simulink library "VariableOrderDifferentialEquationsToolbox"  (R2020a)
settings: Solver=VariableStepAuto  StartTime=0.0  StopTime=10.0  RelTol=1e-3
(part 3 of 3)

== matlab function VariableOrderDifferentialEquationsToolbox/GL FVOPID - Type A/integralErrorDependentSubsystem/Integral Error Depenent Order ==
  data: e input; y output; errorValuesVector input; orderValuesVector input
function y = integralOrderFunction(e, errorValuesVector, orderValuesVector)
    y = fvopidToolbox.utils.getOrderValue(e, errorValuesVector, orderValuesVector);
end

== matlab function VariableOrderDifferentialEquationsToolbox/GL FVOPID - Type A/derivativeRatioDependentSubsystem/Integral Error Depenent Order 2 ==
  data: e input; setpoint input; y output; errorValuesVector input; orderValuesVector input
function y = integralOrderFunction(e, setpoint, errorValuesVector, orderValuesVector)
    y = fvopidToolbox.utils.getOrderValue(e/setpoint, errorValuesVector, orderValuesVector);
end

== matlab function VariableOrderDifferentialEquationsToolbox/GL FVOPID - Type A/integralTimeDependentSubsystem/integralTimeDependentBlock ==
  data: t input; y output; e input
function y = integralTimeDependentMatlabFunction(t, e)
y = 3 * t + 2 * e;
end

== matlab function VariableOrderDifferentialEquationsToolbox/GL FVOPID - Type A/derivativeTimeDependentSubsystem/derivativeTimeDependentBlock ==
  data: t input; y output; e input
function y = derivativeTimeDependentMatlabFunction(t, e)
y = 2*t + e;
end

== matlab function VariableOrderDifferentialEquationsToolbox/GL FVOPID - Type A (external orders)/fvopidOptimized ==
  data: e input; u output; kp input; ki input; kd input; vi input; vd input; h input; N input; saturationEnabled input; saturationLimitLow input; saturationLimitHigh input
function u = fvopidOptimized(e, kp, ki, kd, vi, vd, h, N, saturationEnabled, saturationLimitLow, saturationLimitHigh)
    u = fvopidToolbox.fvopid.fvopidTypeA(e, kp, ki, kd, vi, vd, h, N, saturationEnabled, saturationLimitLow, saturationLimitHigh);
